simulink model "BPP_Plausability"  (R2024b)
settings: Solver=VariableStepAuto  StartTime=0.0  StopTime=5  RelTol=1e-3
libraries: simulink x1
settings Model: Creator=Michele  LastModifiedBy=Michele
settings ConfigComp: CovMetricSettings=dcmwe

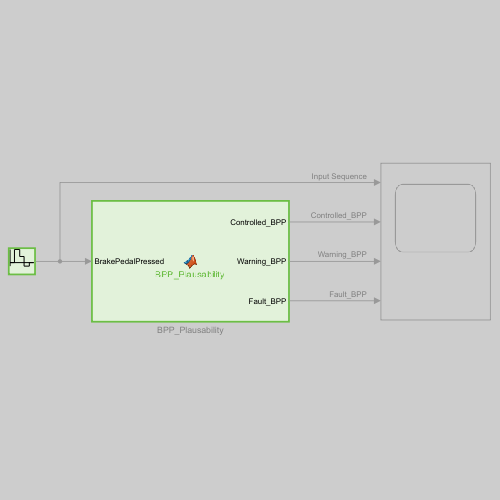
[thumbnail: Simulink's stored preview of the top-level diagram]
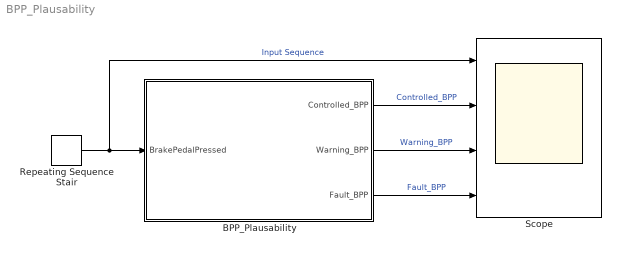
== system BPP_Plausability ==
  BPP_Plausability : MATLAB Function  TreatAsAtomicUnit=on
  Repeating Sequence Stair : simulink/Sources/Repeating Sequence Stair  OutValues=[0 2 1 -0.5 0].'  tsamp=1  OutMin=[]  OutMax=[]  OutDataTypeStr=single  OutputDataTypeScalingMode=single  OutDataType=fixdt('boolean')  ConRadixGroup=Best Precision: Vector-wise  OutScaling=[]
  Scope : Scope  NumInputPorts=4
  wires:
  BPP_Plausability/3(Fault_BPP) -> Scope/4  "Fault_BPP"
  Repeating Sequence Stair/1 -> Scope/1, BPP_Plausability/1(BrakePedalPressed)  "Input Sequence"
  BPP_Plausability/1(Controlled_BPP) -> Scope/2  "Controlled_BPP"
  BPP_Plausability/2(Warning_BPP) -> Scope/3  "Warning_BPP"

== matlab function BPP_Plausability/BPP_Plausability ==
  data: BrakePedalPressed input; Controlled_BPP output; Warning_BPP output Enum: WarningType; Fault_BPP output boolean
function [Controlled_BPP,Warning_BPP,Fault_BPP] = BPP_Plausability(BrakePedalPressed)

Warning_BPP = WarningType(0);
Fault_BPP = boolean(0);
Controlled_BPP = boolean(0);

if (BrakePedalPressed == 0 || BrakePedalPressed == 1) 

    Controlled_BPP = boolean(BrakePedalPressed);
        
else

    Warning_BPP = WarningType(2);
    Fault_BPP = boolean(1);

end
